simulink model "problem3_servo_sim"  (R2019a)
settings: Solver=VariableStepAuto  StartTime=0.0  StopTime=50  RelTol=1e-3
values from neighbouring files (symbols this model uses):
  C = [0.5, 0]    [problem_3.m]
  D_wave = 6    [problem_3.m]
  D_wind = 7    [problem_3.m]
  k_servo = b'*s_inf    [problem_3.m]
  w_n = 2    [problem_3.m]
  x_init = [x1_init(i), x2_init(i)]'    [problem_2.m]    (also in problem_3.m = [ 0.3, 0])
  zeta = 0.4    [problem_3.m]
settings Model: Creator=glitch  LastModifiedBy=glitch

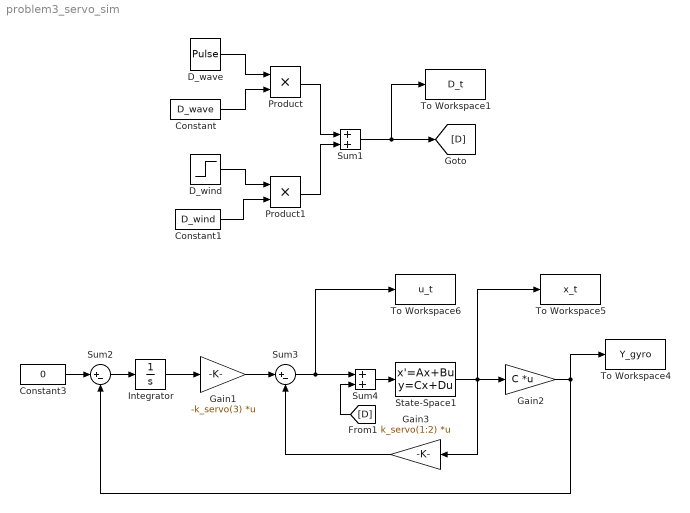
== system problem3_servo_sim ==
  Constant : Constant  Value=D_wave
  Constant1 : Constant  Value=D_wind
  Constant3 : Constant  Value=0
  D_wave : DiscretePulseGenerator  PulseType=Time based  Period=1  PulseWidth=10
  D_wind : Step  Time=10  SampleTime=0
  Gain1 : Gain  Gain=-k_servo(3)  Multiplication=Matrix(K*u)
  Gain2 : Gain  Gain=C  Multiplication=Matrix(K*u)
  Gain3 : Gain  Gain=k_servo(1:2)  Multiplication=Matrix(K*u)
  Integrator : Integrator
  Product : Product
  Product1 : Product
  State-Space1 : StateSpace  A=[0,1; -w_n^2, -2*w_n*zeta]  B=[0; 2*w_n^2]  C=eye(2)  D=[0;0]  InitialCondition=x_init
  Sum1 : Sum
  Sum2 : Sum  Inputs=|+-
  Sum3 : Sum  Inputs=|+-
  Sum4 : Sum
  To Workspace1 : ToWorkspace  VariableName=D_t  SaveFormat=Structure With Time  SampleTime=-1
  To Workspace4 : ToWorkspace  VariableName=Y_gyro  SaveFormat=Structure With Time  SampleTime=-1
  To Workspace5 : ToWorkspace  VariableName=x_t  SaveFormat=Structure With Time  SampleTime=-1
  To Workspace6 : ToWorkspace  VariableName=u_t  SaveFormat=Structure With Time  SampleTime=-1
  wires:
  State-Space1/1 -> Gain2/1, Gain3/1, To Workspace5/1
  Sum4/1 -> State-Space1/1
  Gain3/1 -> Sum3/2
  [D] -> Sum4/2
  Sum1/1 -> [D], To Workspace1/1
  D_wave/1 -> Product/1
  Product/1 -> Sum1/1
  D_wind/1 -> Product1/1
  Constant/1 -> Product/2
  Constant1/1 -> Product1/2
  Product1/1 -> Sum1/2
  Constant3/1 -> Sum2/1
  Gain2/1 -> Sum2/2, To Workspace4/1
  Integrator/1 -> Gain1/1
  Sum2/1 -> Integrator/1
  Gain1/1 -> Sum3/1
  Sum3/1 -> To Workspace6/1, Sum4/1
